simulink model "SEIRv3"  (R2019b)
settings: Solver=VariableStepAuto  StartTime=0.0  StopTime=365  FixedStep=1/24  RelTol=1e-6
settings Model: Creator=Alex  LastModifiedBy=Alex

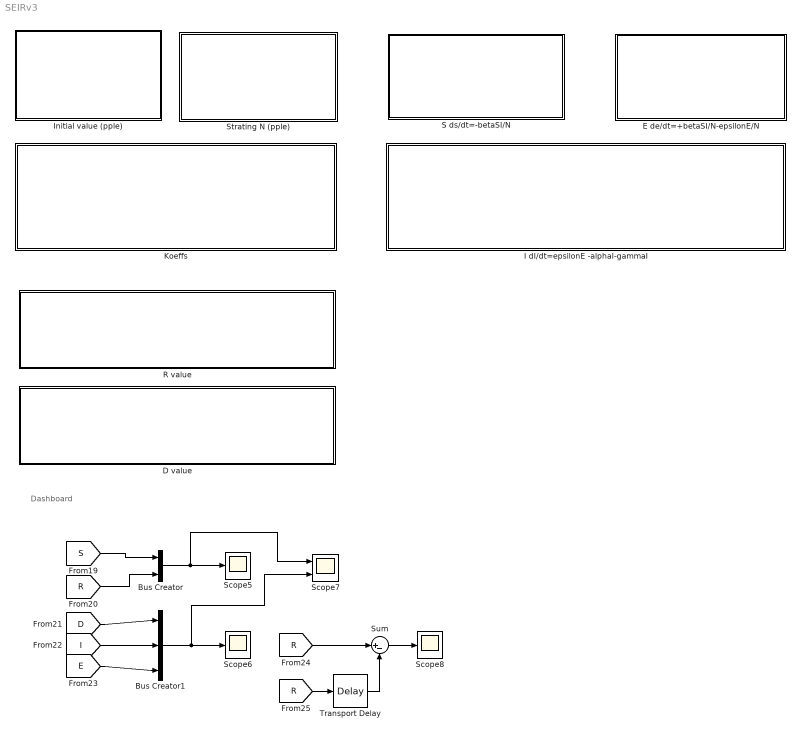
== system SEIRv3 ==
  note: Dashboard
  Bus Creator : BusCreator  Inputs=2
  Bus Creator1 : BusCreator  Inputs=3
  D value : Subsystem
  E de/dt=+betaSI/N-epsilonE/N : Subsystem
  I dI/dt=epsilonE -alphaI-gammaI : Subsystem
  Initial value (pple) : Subsystem
  Koeffs : Subsystem
  R value : Subsystem
  S ds/dt=-betaSI/N : Subsystem
  Scope5 : Scope
  Scope6 : Scope
  Scope7 : Scope  NumInputPorts=2
  Scope8 : Scope
  Strating N (pple) : Subsystem
  Sum : Sum  Inputs=|+-
  Transport Delay : TransportDelay
  wires:
  [S] -> Bus Creator/1
  [R] -> Bus Creator/2
  [D] -> Bus Creator1/1
  [I] -> Bus Creator1/2
  [E] -> Bus Creator1/3
  Bus Creator/1 -> Scope7/1, Scope5/1
  Bus Creator1/1 -> Scope7/2, Scope6/1
  [R] -> Transport Delay/1
  [R] -> Sum/1
  Transport Delay/1 -> Sum/2
  Sum/1 -> Scope8/1

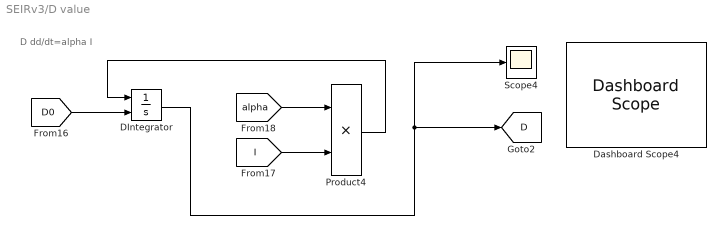
== system SEIRv3/D value ==
  note: D dd/dt=alpha I
  DIntegrator : Integrator  InitialConditionSource=external
  Dashboard Scope4 : DashboardScope  Ymax=150e6
  Product4 : Product  Inputs=**
  Scope4 : Scope
  tag scope: D=global
  wires:
  DIntegrator/1 -> [D], Scope4/1
  [I] -> Product4/2
  [alpha] -> Product4/1
  Product4/1 -> DIntegrator/1
  [D0] -> DIntegrator/2

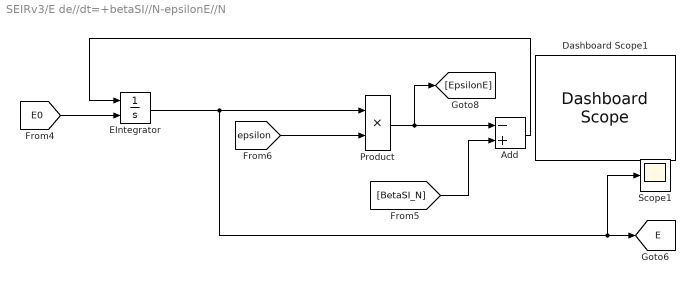
== system SEIRv3/E de//dt=+betaSI//N-epsilonE//N ==
  Add : Sum  Inputs=-+
  Dashboard Scope1 : DashboardScope  Ymax=150e6
  EIntegrator : Integrator  InitialConditionSource=external
  Product : Product  Inputs=**
  Scope1 : Scope
  tag scope: E=global
  wires:
  EIntegrator/1 -> Scope1/1, [E], Product/1
  [BetaSI_N] -> Add/2
  Add/1 -> EIntegrator/1
  [epsilon] -> Product/2
  Product/1 -> [EpsilonE], Add/1
  [E0] -> EIntegrator/2

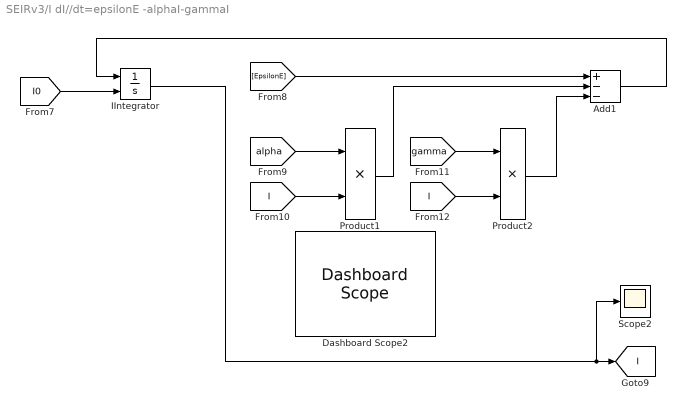
== system SEIRv3/I dI//dt=epsilonE -alphaI-gammaI ==
  Add1 : Sum  Inputs=+--
  Dashboard Scope2 : DashboardScope  Ymax=150e6
  IIntegrator : Integrator  InitialConditionSource=external
  Product1 : Product  Inputs=**
  Product2 : Product  Inputs=**
  Scope2 : Scope
  tag scope: I=global
  wires:
  [gamma] -> Product2/1
  Product2/1 -> Add1/3
  [EpsilonE] -> Add1/1
  [alpha] -> Product1/1
  Product1/1 -> Add1/2
  IIntegrator/1 -> [I], Scope2/1
  [I] -> Product1/2
  Add1/1 -> IIntegrator/1
  [I] -> Product2/2
  [I0] -> IIntegrator/2

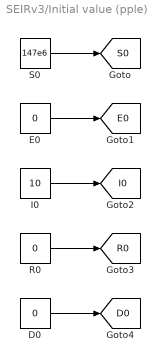
== system SEIRv3/Initial value (pple) ==
  D0 : Constant  Value=0
  E0 : Constant  Value=0
  I0 : Constant  Value=10
  R0 : Constant  Value=0
  S0 : Constant  Value=147e6
  tag scope: D0=global, E0=global, I0=global, R0=global, S0=global
  wires:
  S0/1 -> [S0]
  I0/1 -> [I0]
  D0/1 -> [D0]
  E0/1 -> [E0]
  R0/1 -> [R0]

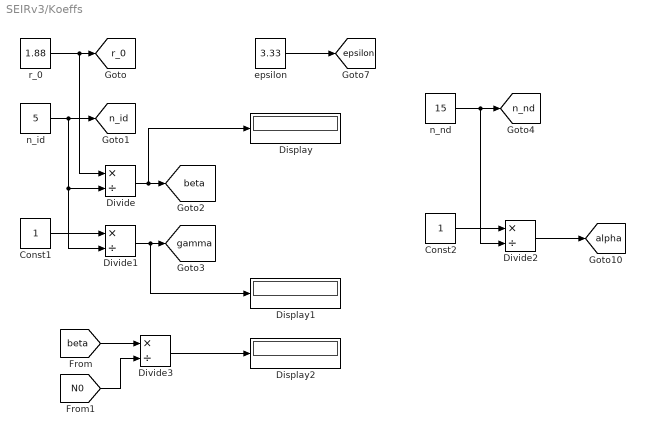
== system SEIRv3/Koeffs ==
  Const1 : Constant
  Const2 : Constant
  Display : Display
  Display1 : Display
  Display2 : Display
  Divide{,1..3} (4 alike) : Product  Inputs=*/
  epsilon : Constant  Value=3.33
  n_id : Constant  Value=5
  n_nd : Constant  Value=15
  r_0 : Constant  Value=1.88
  tag scope: alpha=global, beta=global, epsilon=global, gamma=global, n_id=global, n_nd=global, r_0=global
  wires:
  r_0/1 -> Divide/1, [r_0]
  Divide1/1 -> Display1/1, [gamma]
  n_id/1 -> Divide1/2, Divide/2, [n_id]
  Divide/1 -> Display/1, [beta]
  Const1/1 -> Divide1/1
  epsilon/1 -> [epsilon]
  Const2/1 -> Divide2/1
  Divide2/1 -> [alpha]
  n_nd/1 -> [n_nd], Divide2/2
  [beta] -> Divide3/1
  [N0] -> Divide3/2
  Divide3/1 -> Display2/1

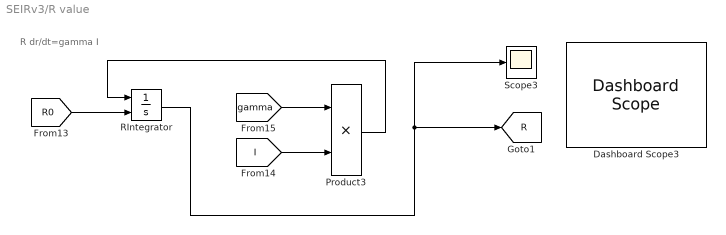
== system SEIRv3/R value ==
  note: R dr/dt=gamma I
  Dashboard Scope3 : DashboardScope  Ymax=150e6
  Product3 : Product  Inputs=**
  RIntegrator : Integrator  InitialConditionSource=external
  Scope3 : Scope
  tag scope: R=global
  wires:
  Product3/1 -> RIntegrator/1
  [I] -> Product3/2
  [R0] -> RIntegrator/2
  [gamma] -> Product3/1
  RIntegrator/1 -> Scope3/1, [R]

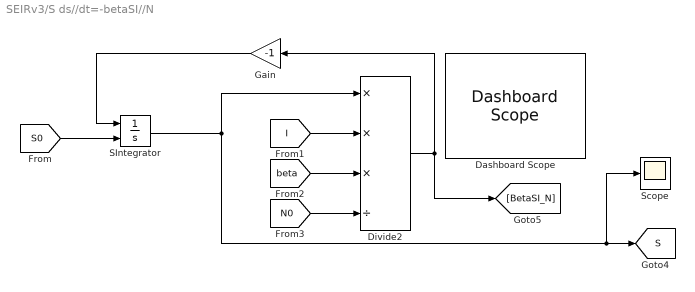
== system SEIRv3/S ds//dt=-betaSI//N ==
  Dashboard Scope : DashboardScope  Ymax=150e6
  Divide2 : Product  Inputs=***/
  Gain : Gain  Gain=-1
  SIntegrator : Integrator  InitialConditionSource=external
  Scope : Scope
  tag scope: S=global
  wires:
  Divide2/1 -> [BetaSI_N], Gain/1
  SIntegrator/1 -> Scope/1, [S], Divide2/1
  [N0] -> Divide2/4
  [beta] -> Divide2/3
  [I] -> Divide2/2
  Gain/1 -> SIntegrator/1
  [S0] -> SIntegrator/2

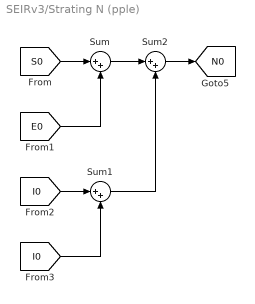
== system SEIRv3/Strating N (pple) ==
  Sum : Sum  Inputs=|++
  Sum1 : Sum  Inputs=|++
  Sum2 : Sum  Inputs=|++
  tag scope: N0=global
  wires:
  [I0] -> Sum1/1
  [S0] -> Sum/1
  [E0] -> Sum/2
  [I0] -> Sum1/2
  Sum2/1 -> [N0]
  Sum1/1 -> Sum2/2
  Sum/1 -> Sum2/1
